simulink model "Braking_dynamics_model"  (R2025a)
settings: Solver=FixedStepAuto  StartTime=0.0  StopTime=3  FixedStep=0.01  RelTol=1e-3
values from neighbouring files (symbols this model uses):
  a = 1.8    [Longitudinal_Braking_parameters.m]
  A = 1.25    [Longitudinal_Braking_parameters.m]
  a1 = -1e-5    (= -1e-05)    [Longitudinal_Braking_parameters.m]
  a2 = 1.25    [Longitudinal_Braking_parameters.m]
  b = L-a    (= 1.7)    [Longitudinal_Braking_parameters.m]
  B = 4.1576    [Longitudinal_Braking_parameters.m]
  balance = 0.65    [Longitudinal_Braking_parameters.m]    (also in Run_Braking_Aero_Comparison.m)
  C = 1.7180    (= 1.718)    [Longitudinal_Braking_parameters.m]
  cd = 0.4    [Longitudinal_Braking_parameters.m]
  cz = 1    [Longitudinal_Braking_parameters.m]
  g = 9.81    [Longitudinal_Braking_parameters.m]
  h = 0.2    [Longitudinal_Braking_parameters.m]
  Iwheel = 0.9    [Longitudinal_Braking_parameters.m]
  L = 3.5    [Longitudinal_Braking_parameters.m]
  m = 850    [Longitudinal_Braking_parameters.m]
  r = 0.375    [Longitudinal_Braking_parameters.m]
  rbrake = 3800    [Longitudinal_Braking_parameters.m]
  rho = 1.225    [Longitudinal_Braking_parameters.m]
settings Model: Creator=g.m.morjaria  LastModifiedBy=g.m.morjaria

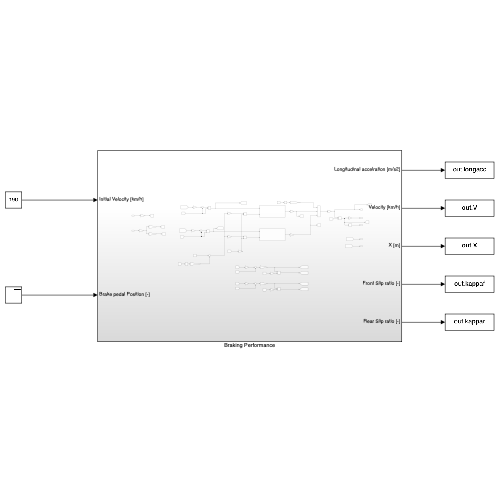
[thumbnail: Simulink's stored preview of the top-level diagram]
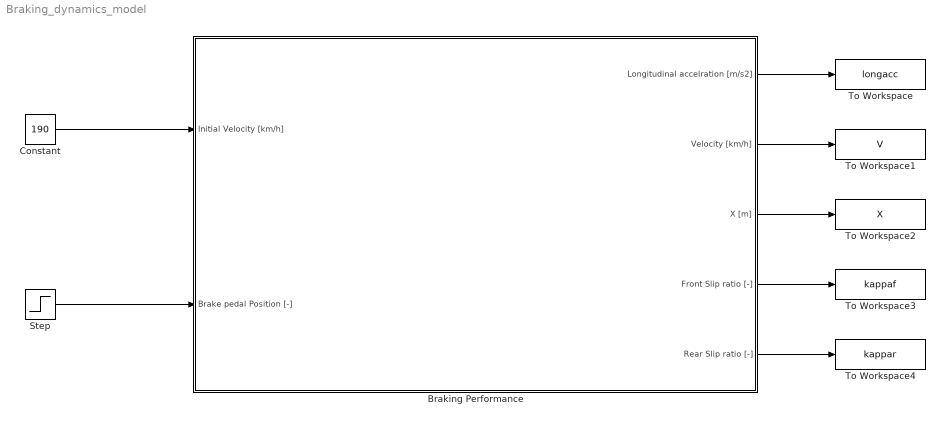
== system Braking_dynamics_model ==
  Braking Performance : Subsystem
  Constant : Constant  Value=190
  Step : Step  After=0.85  SampleTime=0
  To Workspace : ToWorkspace  VariableName=longacc  SaveFormat=Timeseries  SampleTime=-1
  To Workspace1 : ToWorkspace  VariableName=V  SaveFormat=Timeseries  SampleTime=-1
  To Workspace2 : ToWorkspace  VariableName=X  SaveFormat=Timeseries  SampleTime=-1
  To Workspace3 : ToWorkspace  VariableName=kappaf  SaveFormat=Timeseries  SampleTime=-1
  To Workspace4 : ToWorkspace  VariableName=kappar  SaveFormat=Timeseries  SampleTime=-1
  wires:
  Braking Performance/1(Longitudinal accelration [m/s2]) -> To Workspace/1
  Braking Performance/2(Velocity [km/h]) -> To Workspace1/1
  Braking Performance/3(X [m]) -> To Workspace2/1
  Braking Performance/4(Front Slip ratio [-]) -> To Workspace3/1
  Braking Performance/5(Rear Slip ratio [-]) -> To Workspace4/1
  Constant/1 -> Braking Performance/1(Initial Velocity [km/h])
  Step/1 -> Braking Performance/2(Brake pedal Position [-])

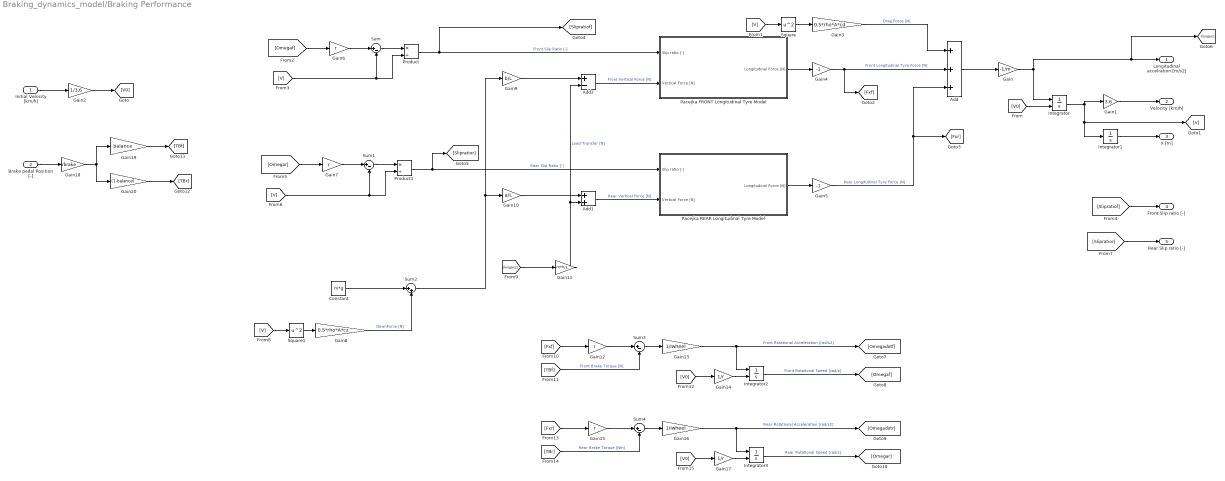
== system Braking_dynamics_model/Braking Performance ==
  Initial Velocity [km/h] : Inport
  Brake pedal Position [-] : Inport  Port=2
  Add : Sum  Inputs=+++
  Add1 : Sum
  Add2 : Sum  Inputs=+-
  Constant : Constant  Value=m*g
  Gain : Gain  Gain=-1/m
  Gain1 : Gain  Gain=3.6
  Gain10 : Gain  Gain=a/L
  Gain11 : Gain  Gain=m*h/L
  Gain{6..7,12,15} (4 alike) : Gain  Gain=r
  Gain13 : Gain  Gain=1/Iwheel
  Gain14 : Gain  Gain=1/r
  Gain16 : Gain  Gain=1/Iwheel
  Gain17 : Gain  Gain=1/r
  Gain18 : Gain  Gain=rbrake
  Gain19 : Gain  Gain=balance
  Gain2 : Gain  Gain=1/3.6
  Gain20 : Gain  Gain=(1-balance)
  Gain3 : Gain  Gain=0.5*rho*A*cd
  Gain4 : Gain  Gain=-1
  Gain5 : Gain  Gain=-1
  Gain8 : Gain  Gain=0.5*rho*A*cz
  Gain9 : Gain  Gain=b/L
  Integrator : Integrator  InitialConditionSource=external
  Integrator1 : Integrator
  Integrator2 : Integrator  InitialConditionSource=external
  Integrator3 : Integrator  InitialConditionSource=external
  Pacejka FRONT Longitudinal Tyre Model : Subsystem
  Pacejka REAR Longitudinal Tyre Model : Subsystem
  Product : Product  Inputs=*/
  Product1 : Product  Inputs=*/
  Square : Math  Operator=square
  Square1 : Math  Operator=square
  Sum{,1,3..4} (4 alike) : Sum  Inputs=|+-
  Sum2 : Sum  Inputs=|++
  Longitudinal accelration [m/s2] : Outport
  Velocity [km/h] : Outport  Port=2
  X [m] : Outport  Port=3
  Front Slip ratio [-] : Outport  Port=4
  Rear Slip ratio [-] : Outport  Port=5
  wires:
  Gain/1 -> [longacc], Longitudinal accelration [m/s2]/1, Integrator/1
  Integrator1/1 -> X [m]/1
  Gain1/1 -> Velocity [km/h]/1
  Integrator/1 -> Gain1/1, [V], Integrator1/1
  Initial Velocity [km/h]/1 -> Gain2/1
  Gain2/1 -> [V0]
  [V0] -> Integrator/2
  Add/1 -> Gain/1
  [V] -> Square/1
  Square/1 -> Gain3/1
  Gain3/1 -> Add/1  "Drag Force [N]"
  Pacejka FRONT Longitudinal Tyre Model/1(Longitudinal Force [N]) -> Gain4/1
  Gain4/1 -> [Fxf], Add/2  "Front Longitudinal Tyre Force [N]"
  Pacejka REAR Longitudinal Tyre Model/1(Longitudinal Force [N]) -> Gain5/1
  Gain5/1 -> [Fxr], Add/3  "Rear Longitudinal Tyre Force [N]"
  [Omegaf] -> Gain6/1
  Gain6/1 -> Sum/1
  [V] -> Sum/2, Product/2
  Sum/1 -> Product/1
  Product/1 -> [Slipratiof], Pacejka FRONT Longitudinal Tyre Model/1(Slip ratio [-])  "Front Slip Ratio [-]"
  [Slipratiof] -> Front Slip ratio [-]/1
  Product1/1 -> Pacejka REAR Longitudinal Tyre Model/1(Slip ratio [-]), [Slipratior]  "Rear Slip Ratio [-]"
  Sum1/1 -> Product1/1
  [V] -> Product1/2, Sum1/2
  Gain7/1 -> Sum1/1
  [Omegar] -> Gain7/1
  [Slipratior] -> Rear Slip ratio [-]/1
  Square1/1 -> Gain8/1
  [V] -> Square1/1
  Constant/1 -> Sum2/1
  Gain8/1 -> Sum2/2  "DownForce [N]"
  Sum2/1 -> Gain10/1, Gain9/1
  Add1/1 -> Pacejka REAR Longitudinal Tyre Model/2(Vertical Force [N])  "Rear Vertical Force [N]"
  Gain10/1 -> Add1/1
  Gain9/1 -> Add2/1
  Add2/1 -> Pacejka FRONT Longitudinal Tyre Model/2(Vertical Force [N])  "Front Vertical Force [N]"
  [longacc] -> Gain11/1
  Gain11/1 -> Add1/2, Add2/2  "Load Transfer [N]"
  Sum3/1 -> Gain13/1
  [Fxf] -> Gain12/1
  [TBf] -> Sum3/2  "Front Brake Torque [N]"
  Gain12/1 -> Sum3/1
  Gain13/1 -> Integrator2/1, [Omegadotf]  "Front Rotational Acceleration [rad/s2]"
  Integrator2/1 -> [Omegaf]  "Front Rotational Speed [rad/s]"
  Gain14/1 -> Integrator2/2
  [V0] -> Gain14/1
  [V0] -> Gain17/1
  Gain17/1 -> Integrator3/2
  Integrator3/1 -> [Omegar]  "Rear Rotational Speed [rad/s]"
  Gain16/1 -> [Omegadotr], Integrator3/1  "Rear Rotational Acceleration [rad/s2]"
  Gain15/1 -> Sum4/1
  [TBr] -> Sum4/2  "Rear Brake Torque [Nm]"
  [Fxr] -> Gain15/1
  Sum4/1 -> Gain16/1
  Brake pedal Position [-]/1 -> Gain18/1
  Gain18/1 -> Gain19/1, Gain20/1
  Gain20/1 -> [TBr]
  Gain19/1 -> [TBf]

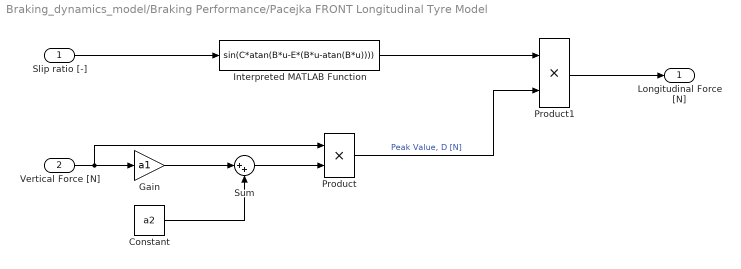
== system Braking_dynamics_model/Braking Performance/Pacejka FRONT Longitudinal Tyre Model ==
  Slip ratio [-] : Inport
  Vertical Force [N] : Inport  Port=2
  Constant : Constant  Value=a2
  Gain : Gain  Gain=a1
  Interpreted MATLAB Function : MATLABFcn  MATLABFcn=sin(C*atan(B*u-E*(B*u-atan(B*u))))
  Product : Product
  Product1 : Product
  Sum : Sum  Inputs=|++
  Longitudinal Force [N] : Outport
  wires:
  Vertical Force [N]/1 -> Product/1, Gain/1
  Gain/1 -> Sum/1
  Constant/1 -> Sum/2
  Sum/1 -> Product/2
  Product/1 -> Product1/2  "Peak Value, D [N]"
  Slip ratio [-]/1 -> Interpreted MATLAB Function/1
  Interpreted MATLAB Function/1 -> Product1/1
  Product1/1 -> Longitudinal Force [N]/1

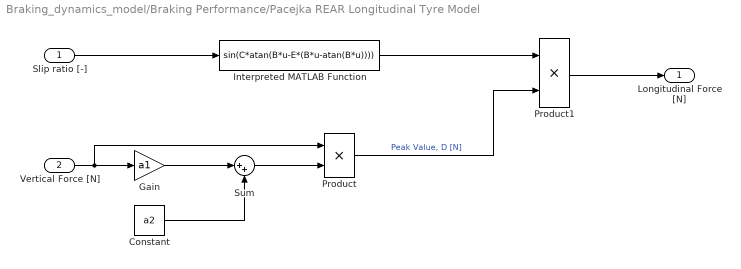
== system Braking_dynamics_model/Braking Performance/Pacejka REAR Longitudinal Tyre Model ==
  Slip ratio [-] : Inport
  Vertical Force [N] : Inport  Port=2
  Constant : Constant  Value=a2
  Gain : Gain  Gain=a1
  Interpreted MATLAB Function : MATLABFcn  MATLABFcn=sin(C*atan(B*u-E*(B*u-atan(B*u))))
  Product : Product
  Product1 : Product
  Sum : Sum  Inputs=|++
  Longitudinal Force [N] : Outport
  wires:
  Product1/1 -> Longitudinal Force [N]/1
  Interpreted MATLAB Function/1 -> Product1/1
  Slip ratio [-]/1 -> Interpreted MATLAB Function/1
  Product/1 -> Product1/2  "Peak Value, D [N]"
  Sum/1 -> Product/2
  Constant/1 -> Sum/2
  Gain/1 -> Sum/1
  Vertical Force [N]/1 -> Gain/1, Product/1
